simulink model "QPSK_complete3"  (R2016b)
settings: Solver=VariableStepAuto  StartTime=0.0  StopTime=(12+133)*8  RelTol=1e-3
undefined symbols (not defined in the file or in its folder): jsin, K1, K2, rcosine
libraries: dspsigops x2, dspstat3 x1, dspsrcs4 x1, simulink x1
settings Model: Creator=colttom  LastModifiedBy=colttom

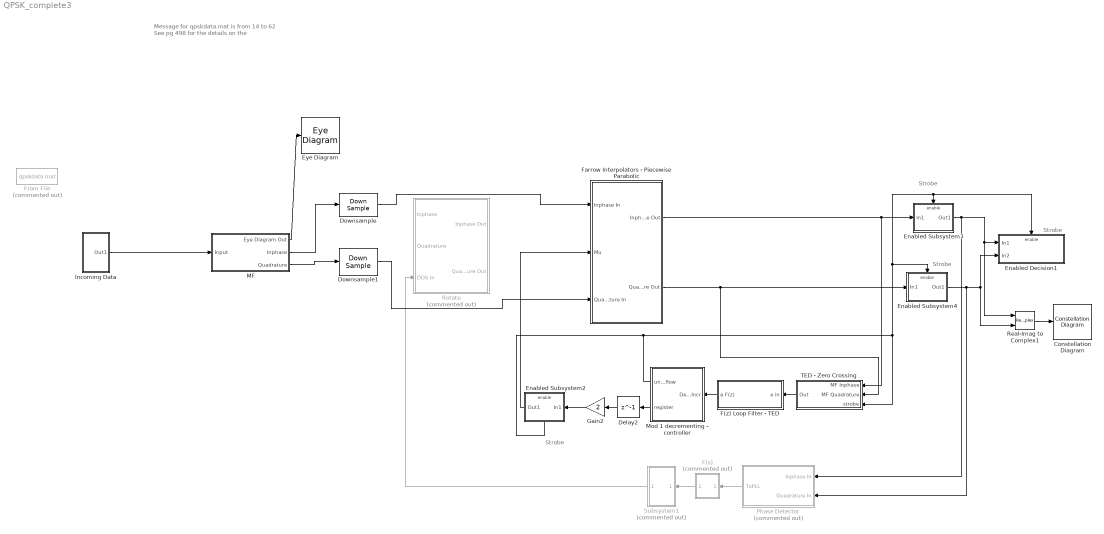
== system QPSK_complete3 ==
  note: Strobe
  note: Strobe
  note: Strobe
  note: Strobe
  note: Message for qpskdata.mat is from 14 to 62
      |
      | See pg 498 for the details on the
  Constellation Diagram : ConstellationDiagram
  Delay2 : Delay  DelayLength=1
  Downsample : DownSample  N=16/2  phase=7  InputProcessing=Inherited (this choice will be removed - see release notes)  RateOptions=Allow multirate processing
  Downsample1 : DownSample  N=16/2  phase=7  InputProcessing=Inherited (this choice will be removed - see release notes)  RateOptions=Allow multirate processing
  Enabled Decision1 : Subsystem  TreatAsAtomicUnit=on
  Enabled Subsystem2 : Subsystem  TreatAsAtomicUnit=on
  Enabled Subsystem3 : Subsystem  TreatAsAtomicUnit=on
  Enabled Subsystem4 : Subsystem  TreatAsAtomicUnit=on
  Eye Diagram : EyeDiagram
  F(s) : Subsystem  Commented=on
  F(z) Loop Filter - TED : Subsystem
  Farrow Interpolators - Piecewise Parabolic : Subsystem
  From File : FromFile  Commented=on  FileName=qpskdata.mat  SampleTime=1
  Gain2 : Gain  Gain=2
  Incoming Data : Subsystem
  MF : Subsystem
  Mod 1 decrementing - controller : Subsystem
  Phase Detector : Subsystem  Commented=on
  Real-Imag to Complex1 : RealImagToComplex
  Rotate : Subsystem  Commented=on
  Subsystem1 : Subsystem  Commented=on
  TED - Zero Crossing : Subsystem
  wires:
  F(z) Loop Filter - TED/1(e F(z)) -> Mod 1 decrementing - controller/1(Delta Incr)
  Mod 1 decrementing - controller/2(register) -> Delay2/1
  Delay2/1 -> Gain2/1
  Gain2/1 -> Enabled Subsystem2/1(In1)
  Mod 1 decrementing - controller/1(underflow) -> Enabled Decision1/Enable, Enabled Subsystem3/Enable, Enabled Subsystem4/Enable, TED - Zero Crossing/3(strobe), Enabled Subsystem2/Enable
  Real-Imag to Complex1/1 -> Constellation Diagram/1
  Enabled Subsystem3/1(Out1) -> Phase Detector/1(Inphase In), Real-Imag to Complex1/1, Enabled Decision1/1(In1)
  Enabled Subsystem4/1(Out1) -> Phase Detector/2(Quadrature In), Enabled Decision1/2(In2), Real-Imag to Complex1/2
  TED - Zero Crossing/1(Out) -> F(z) Loop Filter - TED/1(e in)
  Incoming Data/1(Out1) -> MF/1(Input)
  MF/1(Eye Diagram Out) -> Eye Diagram/1
  MF/2(Inphase) -> Downsample/1
  MF/3(Quadrature) -> Downsample1/1
  Farrow Interpolators - Piecewise Parabolic/2(Quadrature Out) -> TED - Zero Crossing/2(MF Quadrature), Enabled Subsystem4/1(In1)
  Farrow Interpolators - Piecewise Parabolic/1(Inphase Out) -> TED - Zero Crossing/1(MF Inphase), Enabled Subsystem3/1(In1)
  Enabled Subsystem2/1(Out1) -> Farrow Interpolators - Piecewise Parabolic/2(Mu)
  F(s)/1(Out1) -> Subsystem1/1(In1)
  Subsystem1/1(Out1) -> Rotate/3(DDS In)
  Phase Detector/1(ToPLL) -> F(s)/1(In1)
  Downsample/1 -> Farrow Interpolators - Piecewise Parabolic/1(Inphase In)
  Downsample1/1 -> Farrow Interpolators - Piecewise Parabolic/3(Quadrature In)

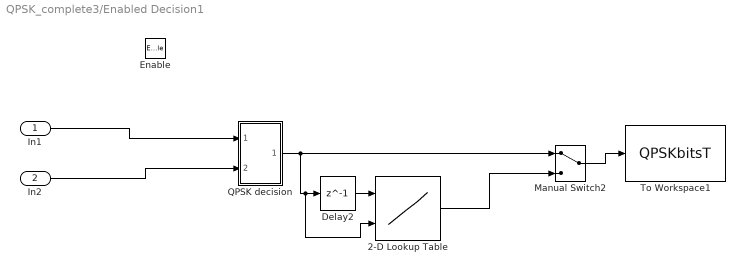
== system QPSK_complete3/Enabled Decision1 ==
  In1 : Inport
  In2 : Inport  Port=2
  Enable : EnablePort
  2-D Lookup Table : Lookup_n-D  BreakpointsForDimension1=[0:3]  BreakpointsForDimension2=[0:3]  Table=[0 1 2 3; 2 0 3 1; 1 3 0 2;3 2 1 0]  InternalRulePriority=Speed  RndMeth=Simplest  InputSameDT=on
  Delay2 : Delay  DelayLength=1
  Manual Switch2 : ManualSwitch
  "QPSK decision " : Subsystem
  To Workspace1 : ToWorkspace  VariableName=QPSKbitsT  SampleTime=-1
      settings: Save2DSignal=2-D array (concatenate along first dimension)
  wires:
  In1/1 -> "QPSK decision "/1(In1)
  In2/1 -> "QPSK decision "/2(In2)
  "QPSK decision "/1(Out1) -> 2-D Lookup Table/2, Delay2/1, Manual Switch2/1
  2-D Lookup Table/1 -> Manual Switch2/2
  Delay2/1 -> 2-D Lookup Table/1
  Manual Switch2/1 -> To Workspace1/1

== system QPSK_complete3/Enabled Subsystem2 ==
  In1 : Inport
  Enable : EnablePort
  Out1 : Outport
  wires:
  In1/1 -> Out1/1

== system QPSK_complete3/Enabled Subsystem3 ==
  In1 : Inport
  Enable : EnablePort
  Out1 : Outport
  wires:
  In1/1 -> Out1/1

== system QPSK_complete3/Enabled Subsystem4 ==
  In1 : Inport
  Enable : EnablePort
  Out1 : Outport
  wires:
  In1/1 -> Out1/1

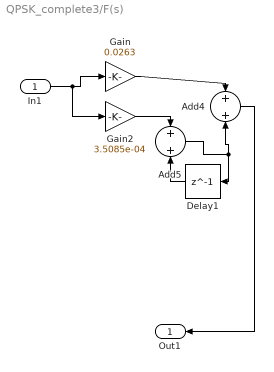
== system QPSK_complete3/F(s) ==
  In1 : Inport
  Add4 : Sum
  Add5 : Sum
  Delay1 : Delay  DelayLength=1
  Gain : Gain  Gain=0.0263
  Gain2 : Gain  Gain=3.5085e-04
  Out1 : Outport
  wires:
  Gain/1 -> Add4/1
  Delay1/1 -> Add5/2
  Add5/1 -> Delay1/1, Add4/2
  Gain2/1 -> Add5/1
  Add4/1 -> Out1/1
  In1/1 -> Gain2/1, Gain/1

== system QPSK_complete3/F(z) Loop Filter - TED ==
  e in : Inport
  Discrete Filter : DiscreteFilter  Numerator=[(K1+K2) -K1]  Denominator=[1 -1]
  e F(z) : Outport
  wires:
  e in/1 -> Discrete Filter/1
  Discrete Filter/1 -> e F(z)/1

== system QPSK_complete3/Farrow Interpolators - Piecewise Parabolic ==
  Inphase In : Inport
  Mu : Inport  Port=2
  Quadrature In : Inport  Port=3
  Interpolation Filter2 : Subsystem
  Interpolation Filter3 : Subsystem
  Inphase Out : Outport
  Quadrature Out : Outport  Port=2
  wires:
  Inphase In/1 -> Interpolation Filter2/1(MF In)
  Quadrature In/1 -> Interpolation Filter3/1(MF In)
  Interpolation Filter2/1(Out) -> Inphase Out/1
  Interpolation Filter3/1(Out) -> Quadrature Out/1
  Mu/1 -> Interpolation Filter2/2(mu), Interpolation Filter3/2(mu)

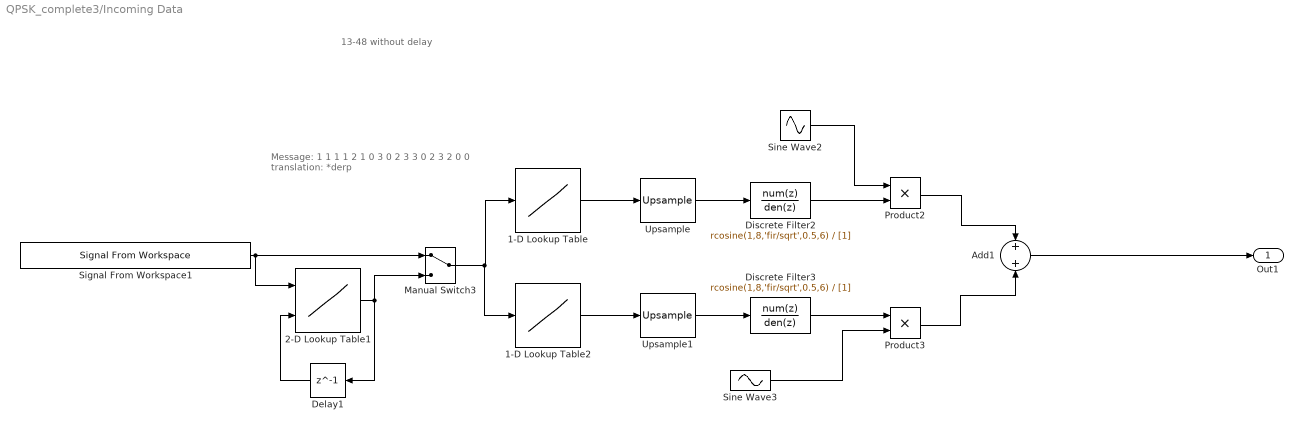
== system QPSK_complete3/Incoming Data ==
  note: 13-48 without delay
  note: Message: 1 1 1 1 2 1 0 3 0 2 3 3 0 2 3 2 0 0
      | translation: *derp
  1-D Lookup Table : Lookup_n-D  NumberOfTableDimensions=1  BreakpointsForDimension1=[0 1 2 3]  Table=[1 -1 1 -1]*3/sqrt(2)  InternalRulePriority=Speed  RndMeth=Simplest  InputSameDT=on
  1-D Lookup Table2 : Lookup_n-D  NumberOfTableDimensions=1  BreakpointsForDimension1=[0 1 2 3]  Table=[1 1 -1 -1]*3/sqrt(2)  InternalRulePriority=Speed  RndMeth=Simplest  InputSameDT=on
  2-D Lookup Table1 : Lookup_n-D  BreakpointsForDimension1=[0:3]  BreakpointsForDimension2=[0:3]  Table=[0 1 2 3;1 3 0 2;2 0 3 1;3 2 1 0]  InternalRulePriority=Speed  RndMeth=Simplest  InputSameDT=on
  Add1 : Sum
  Delay1 : Delay  DelayLength=1
  Discrete Filter2 : DiscreteFilter  Numerator=rcosine(1,8,'fir/sqrt',0.5,6)  Denominator=[1]
  Discrete Filter3 : DiscreteFilter  Numerator=rcosine(1,8,'fir/sqrt',0.5,6)  Denominator=[1]
  Manual Switch3 : ManualSwitch
  Product2 : Product
  Product3 : Product
  Signal From Workspace1 : dspsrcs4/Signal From Workspace  X=[1 2 3 0 0 2 3 1 3 2 1 0 3 2 0 2 0 1 4 2 3 1 0 2 3 1 2 3 0 3 2 1 2 3 0 2 3 3 1 2 3 1 2 3 1 2 3 1 2 1 2 1 2 2 1 2 1 2 1 2 1 2 1 2 1 2 1 2 1 2 1 0 0 3 2 0 1 2 0 1 3 2 3 1 1 1 1 1 0 0 0 1 1 0 0 1 1 1 1 2 1 0 3 0 2 3 3 0 2 3 2 0 0]  Ts=8  nsamps=1  OutputAfterFinalValue=Setting to zero  ignoreOrWarnInputAndFrameLengths=off  OutputFrames=off
  Sine Wave2 : Sin  SineType=Sample based  Amplitude=sqrt(2)  Frequency=2*pi/4  Phase=pi/2  SampleTime=.5
  Sine Wave3 : Sin  SineType=Sample based  Amplitude=-sqrt(2)  Frequency=2*pi/4  SampleTime=.5
  Upsample : dspsigops/Upsample  N=16  phase=0  InputProcessing=Inherited (this choice will be removed - see release notes)  RateOptions=Allow multirate processing  ic=0  mode=Unused parameter value
  Upsample1 : dspsigops/Upsample  N=16  phase=0  InputProcessing=Inherited (this choice will be removed - see release notes)  RateOptions=Allow multirate processing  ic=0  mode=Unused parameter value
  Out1 : Outport
  wires:
  Upsample1/1 -> Discrete Filter3/1
  Discrete Filter2/1 -> Product2/2
  Sine Wave2/1 -> Product2/1
  Discrete Filter3/1 -> Product3/1
  Sine Wave3/1 -> Product3/2
  Product3/1 -> Add1/2
  Product2/1 -> Add1/1
  Add1/1 -> Out1/1
  1-D Lookup Table/1 -> Upsample/1
  1-D Lookup Table2/1 -> Upsample1/1
  Upsample/1 -> Discrete Filter2/1
  2-D Lookup Table1/1 -> Delay1/1, Manual Switch3/2
  Delay1/1 -> 2-D Lookup Table1/2
  Signal From Workspace1/1 -> Manual Switch3/1, 2-D Lookup Table1/1
  Manual Switch3/1 -> 1-D Lookup Table2/1, 1-D Lookup Table/1

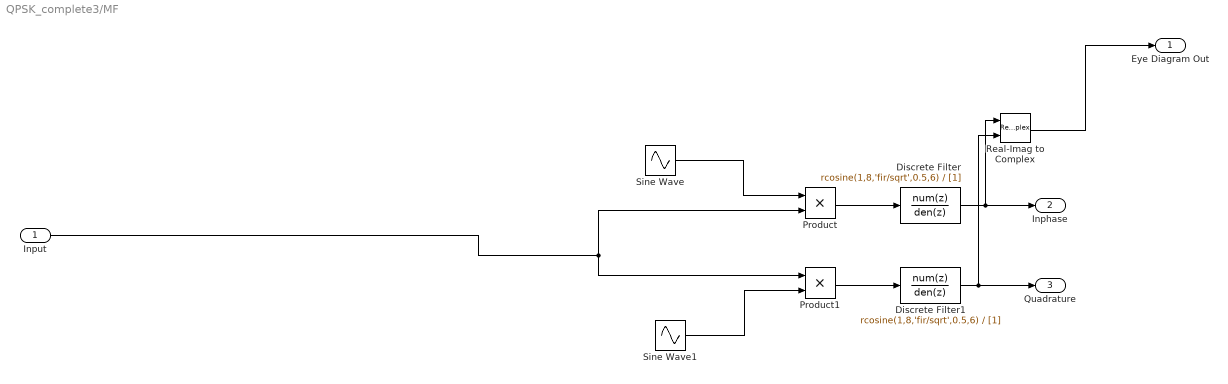
== system QPSK_complete3/MF ==
  Input : Inport
  Discrete Filter : DiscreteFilter  Numerator=rcosine(1,8,'fir/sqrt',0.5,6)  Denominator=[1]
  Discrete Filter1 : DiscreteFilter  Numerator=rcosine(1,8,'fir/sqrt',0.5,6)  Denominator=[1]
  Product : Product
  Product1 : Product
  Real-Imag to Complex : RealImagToComplex
  Sine Wave : Sin  Amplitude=sqrt(2)  Frequency=2*pi/4  Phase=pi/2  SampleTime=.5
  Sine Wave1 : Sin  Amplitude=-sqrt(2)  Frequency=2*pi/4  SampleTime=.5
  Eye Diagram Out : Outport
  Inphase : Outport  Port=2
  Quadrature : Outport  Port=3
  wires:
  Input/1 -> Product/2, Product1/1
  Sine Wave1/1 -> Product1/2
  Sine Wave/1 -> Product/1
  Product1/1 -> Discrete Filter1/1
  Product/1 -> Discrete Filter/1
  Discrete Filter/1 -> Inphase/1, Real-Imag to Complex/1
  Discrete Filter1/1 -> Quadrature/1, Real-Imag to Complex/2
  Real-Imag to Complex/1 -> Eye Diagram Out/1

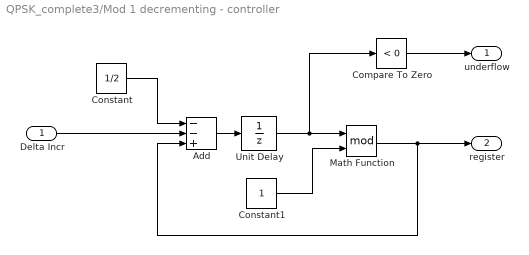
== system QPSK_complete3/Mod 1 decrementing - controller ==
  Delta Incr : Inport
  Add : Sum  Inputs=--+
  Compare To Zero : simulink/Logic and Bit Operations/Compare To Zero  relop=<  OutDataTypeStr=boolean
  Constant : Constant  Value=1/2
  Constant1 : Constant
  Math Function : Math  Operator=mod  SaturateOnIntegerOverflow=on
  Unit Delay : UnitDelay  SampleTime=-1
  underflow : Outport
  register : Outport  Port=2
  wires:
  Delta Incr/1 -> Add/2
  Constant/1 -> Add/1
  Add/1 -> Unit Delay/1
  Constant1/1 -> Math Function/2
  Unit Delay/1 -> Compare To Zero/1, Math Function/1
  Math Function/1 -> Add/3, register/1
  Compare To Zero/1 -> underflow/1

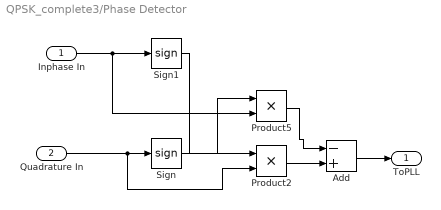
== system QPSK_complete3/Phase Detector ==
  Inphase In : Inport
  Quadrature In : Inport  Port=2
  Add : Sum  Inputs=-+
  Product2 : Product
  Product5 : Product
  Sign : Signum
  Sign1 : Signum
  ToPLL : Outport
  wires:
  Add/1 -> ToPLL/1
  Quadrature In/1 -> Product2/2, Sign/1
  Product5/1 -> Add/1
  Product2/1 -> Add/2
  Inphase In/1 -> Product5/2, Sign1/1
  Sign1/1 -> Product2/1
  Sign/1 -> Product5/1

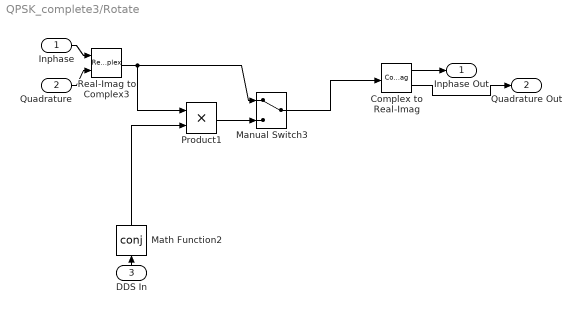
== system QPSK_complete3/Rotate ==
  Inphase : Inport
  Quadrature : Inport  Port=2
  DDS In : Inport  Port=3
  Complex to Real-Imag : ComplexToRealImag
  Manual Switch3 : ManualSwitch
  Math Function2 : Math  Operator=conj  SaturateOnIntegerOverflow=on
  Product1 : Product
  Real-Imag to Complex3 : RealImagToComplex
  Inphase Out : Outport
  Quadrature Out : Outport  Port=2
  wires:
  Real-Imag to Complex3/1 -> Manual Switch3/1, Product1/1
  Math Function2/1 -> Product1/2
  DDS In/1 -> Math Function2/1
  Quadrature/1 -> Real-Imag to Complex3/2
  Inphase/1 -> Real-Imag to Complex3/1
  Complex to Real-Imag/1 -> Inphase Out/1
  Complex to Real-Imag/2 -> Quadrature Out/1
  Manual Switch3/1 -> Complex to Real-Imag/1
  Product1/1 -> Manual Switch3/2

== system QPSK_complete3/Subsystem1 ==
  In1 : Inport
  Add1 : Sum  Inputs=+++
  Constant2 : Constant  Value=0
  Delay : Delay  DelayLength=1
  Gain1 : Gain
  Trigonometric Function : Trigonometry  Operator=cos + jsin
  Out1 : Outport
  wires:
  In1/1 -> Gain1/1
  Constant2/1 -> Add1/1
  Add1/1 -> Delay/1
  Delay/1 -> Trigonometric Function/1, Add1/3
  Gain1/1 -> Add1/2
  Trigonometric Function/1 -> Out1/1

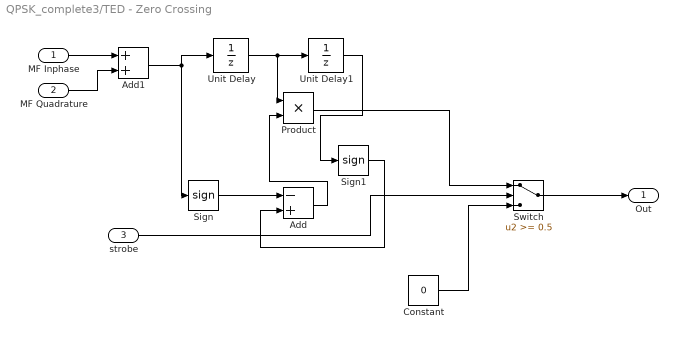
== system QPSK_complete3/TED - Zero Crossing ==
  MF Inphase : Inport
  MF Quadrature : Inport  Port=2
  strobe : Inport  Port=3
  Add : Sum  Inputs=-+
  Add1 : Sum
  Constant : Constant  Value=0
  Product : Product
  Sign : Signum
  Sign1 : Signum
  Switch : Switch  Threshold=0.5  SaturateOnIntegerOverflow=on
  Unit Delay : UnitDelay  SampleTime=-1
  Unit Delay1 : UnitDelay  SampleTime=-1
  Out : Outport
  wires:
  Switch/1 -> Out/1
  Constant/1 -> Switch/3
  strobe/1 -> Switch/2
  Unit Delay/1 -> Product/1, Unit Delay1/1
  Sign/1 -> Add/1
  Add/1 -> Product/2
  Unit Delay1/1 -> Sign1/1
  Sign1/1 -> Add/2
  Product/1 -> Switch/1
  Add1/1 -> Sign/1, Unit Delay/1
  MF Inphase/1 -> Add1/1
  MF Quadrature/1 -> Add1/2

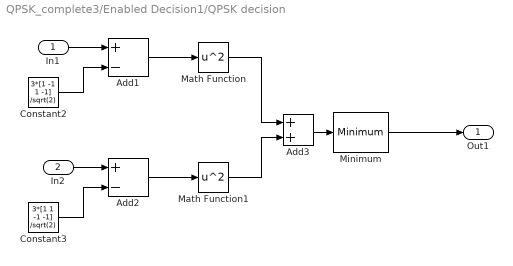
== system QPSK_complete3/Enabled Decision1/QPSK decision  ==
  In1 : Inport
  In2 : Inport  Port=2
  Add1 : Sum  Inputs=+-
  Add2 : Sum  Inputs=+-
  Add3 : Sum
  Constant2 : Constant  Value=3*[1 -1 1 -1] /sqrt(2)
  Constant3 : Constant  Value=3*[1 1 -1 -1] /sqrt(2)
  Math Function : Math  Operator=square  SaturateOnIntegerOverflow=on
  Math Function1 : Math  Operator=square  SaturateOnIntegerOverflow=on
  Minimum : dspstat3/Minimum  operation=minimum  fcn=Index  indexBase=Zero  operateOver=Each column  Dimension=1  InputProcessing=Columns as channels (frame based)  reset=None  roiEnable=off  roiType=Rectangles  roiPortion=Entire ROI  roiOutput=Individual statistics for each ROI  roiFlag=off  roundingMode=Floor  overflowMode=off
  Out1 : Outport
  wires:
  Math Function/1 -> Add3/1
  Math Function1/1 -> Add3/2
  Add3/1 -> Minimum/1
  Minimum/1 -> Out1/1
  Add1/1 -> Math Function/1
  Add2/1 -> Math Function1/1
  Constant3/1 -> Add2/2
  Constant2/1 -> Add1/2
  In1/1 -> Add1/1
  In2/1 -> Add2/1

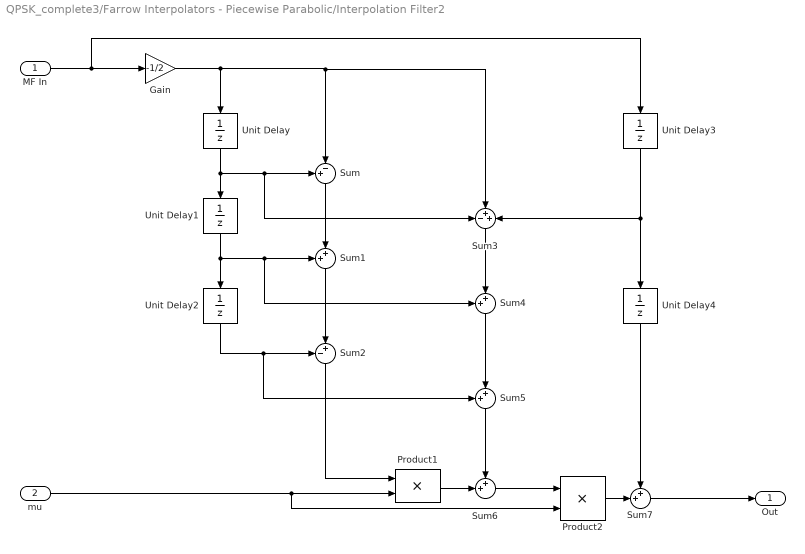
== system QPSK_complete3/Farrow Interpolators - Piecewise Parabolic/Interpolation Filter2 ==
  MF In : Inport
  mu : Inport  Port=2
  Gain : Gain  Gain=-1/2
  Product1 : Product  SaturateOnIntegerOverflow=on  InputSameDT=on  OutDataTypeStr=Inherit: Same as first input
  Product2 : Product  SaturateOnIntegerOverflow=on  InputSameDT=on  OutDataTypeStr=Inherit: Same as first input
  Sum : Sum  Inputs=+-|  SaturateOnIntegerOverflow=on  InputSameDT=on  OutDataTypeStr=Inherit: Same as first input
  Sum{1,4..7} (5 alike) : Sum  Inputs=++|  SaturateOnIntegerOverflow=on  InputSameDT=on  OutDataTypeStr=Inherit: Same as first input
  Sum2 : Sum  Inputs=-+|  SaturateOnIntegerOverflow=on  InputSameDT=on  OutDataTypeStr=Inherit: Same as first input
  Sum3 : Sum  Inputs=-++  SaturateOnIntegerOverflow=on  InputSameDT=on  OutDataTypeStr=Inherit: Same as first input
  Unit Delay{,1..4} (5 alike) : UnitDelay  SampleTime=-1
  Out : Outport
  wires:
  Sum1/1 -> Sum2/2
  Sum/1 -> Sum1/2
  Unit Delay/1 -> Sum3/1, Sum/1, Unit Delay1/1
  Unit Delay1/1 -> Sum4/1, Sum1/1, Unit Delay2/1
  Unit Delay2/1 -> Sum5/1, Sum2/1
  Sum5/1 -> Sum6/1
  Product1/1 -> Sum6/2
  Sum4/1 -> Sum5/2
  Sum3/1 -> Sum4/2
  MF In/1 -> Unit Delay3/1, Gain/1
  Gain/1 -> Unit Delay/1, Sum/2, Sum3/2
  Product2/1 -> Sum7/2
  Unit Delay4/1 -> Sum7/1
  Sum6/1 -> Product2/1
  Sum7/1 -> Out/1
  Unit Delay3/1 -> Sum3/3, Unit Delay4/1
  Sum2/1 -> Product1/1
  mu/1 -> Product2/2, Product1/2

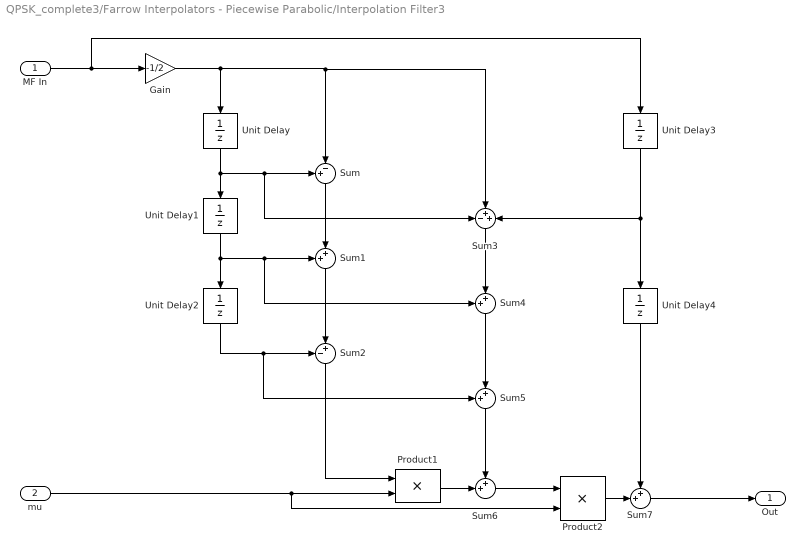
== system QPSK_complete3/Farrow Interpolators - Piecewise Parabolic/Interpolation Filter3 ==
  MF In : Inport
  mu : Inport  Port=2
  Gain : Gain  Gain=-1/2
  Product1 : Product  SaturateOnIntegerOverflow=on  InputSameDT=on  OutDataTypeStr=Inherit: Same as first input
  Product2 : Product  SaturateOnIntegerOverflow=on  InputSameDT=on  OutDataTypeStr=Inherit: Same as first input
  Sum : Sum  Inputs=+-|  SaturateOnIntegerOverflow=on  InputSameDT=on  OutDataTypeStr=Inherit: Same as first input
  Sum{1,4..7} (5 alike) : Sum  Inputs=++|  SaturateOnIntegerOverflow=on  InputSameDT=on  OutDataTypeStr=Inherit: Same as first input
  Sum2 : Sum  Inputs=-+|  SaturateOnIntegerOverflow=on  InputSameDT=on  OutDataTypeStr=Inherit: Same as first input
  Sum3 : Sum  Inputs=-++  SaturateOnIntegerOverflow=on  InputSameDT=on  OutDataTypeStr=Inherit: Same as first input
  Unit Delay{,1..4} (5 alike) : UnitDelay  SampleTime=-1
  Out : Outport
  wires:
  Sum1/1 -> Sum2/2
  Sum/1 -> Sum1/2
  Unit Delay/1 -> Sum3/1, Sum/1, Unit Delay1/1
  Unit Delay1/1 -> Sum4/1, Sum1/1, Unit Delay2/1
  Unit Delay2/1 -> Sum5/1, Sum2/1
  Sum5/1 -> Sum6/1
  Product1/1 -> Sum6/2
  Sum4/1 -> Sum5/2
  Sum3/1 -> Sum4/2
  MF In/1 -> Unit Delay3/1, Gain/1
  Gain/1 -> Unit Delay/1, Sum/2, Sum3/2
  Product2/1 -> Sum7/2
  Unit Delay4/1 -> Sum7/1
  Sum6/1 -> Product2/1
  Sum7/1 -> Out/1
  Unit Delay3/1 -> Sum3/3, Unit Delay4/1
  Sum2/1 -> Product1/1
  mu/1 -> Product2/2, Product1/2
